simulink model "auto_pilot_udp"  (R2022b)
settings: Solver=FixedStepAuto  StartTime=0.0  StopTime=Inf  FixedStep=0.001  RelTol=1e-3  EnableMultiTasking=on
InitFcn:
  | clear mex
model workspace (MAT data in the model file):
  worldsim_instance : object (value not decoded)
values from neighbouring files (symbols this model uses):
  ACC_Adaptive_D = 0    [AutoPilot_parameters.m]    (also in ap_ini_param.mat; ap_initialModel.sldd = 0.0)
  ACC_Adaptive_I = 0    [AutoPilot_parameters.m]    (also in ap_ini_param.mat; ap_initialModel.sldd = 0.0)
  ACC_Adaptive_P = [5 7.5]    [AutoPilot_parameters.m]    (also in ap_ini_param.mat; ap_initialModel.sldd = 5.0 7.5)
  ACC_Classic_I = 5    [AutoPilot_parameters.m]    (also in ap_ini_param.mat; ap_initialModel.sldd = 5.0)
  ACC_Classic_P = 15    [AutoPilot_parameters.m]    (also in ap_ini_param.mat; ap_initialModel.sldd = 15.0)
  ACC_MaxBrake = 50    [AutoPilot_parameters.m]    (also in ap_ini_param.mat; ap_initialModel.sldd = 50.0)
  ACC_MaxThrottle = 130    [AutoPilot_parameters.m]    (also in ap_ini_param.mat = 80; ap_initialModel.sldd = 130.0)
  ACC_Module_Activity_Flag = 1    [AutoPilot_parameters.m]    (also in ap_ini_param.mat; ap_initialModel.sldd = 1.0)
  ACC_Ready_Speed = 30    [AutoPilot_parameters.m]    (also in ap_ini_param.mat; ap_initialModel.sldd = 30.0)
  ACC_SensorMaxDistance = 250    [AutoPilot_parameters.m]    (also in ap_ini_param.mat = 120; ap_initialModel.sldd = 250.0)
  ACC_Speed_Distance_control = 3    [AutoPilot_parameters.m]    (also in ap_ini_param.mat; ap_initialModel.sldd = 3.0)
  ACC_Speed_Distance_Gain = [0.1 0.15 0.2 0.25]    [AutoPilot_parameters.m]    (also in ap_ini_param.mat; ap_initialModel.sldd = 0.1 0.15 0.2 0.25)
  ADAS_Control_Mode = 1    [AutoPilot_parameters.m]    (also in ap_ini_param.mat; ap_initialModel.sldd = 1.0)
  AEB_Alarm_Freq = 5    [AutoPilot_parameters.m]    (also in ap_ini_param.mat; ap_initialModel.sldd = 5.0)
  AEB_Distance_To_Collision_Brake = 5    [AutoPilot_parameters.m]    (also in ap_ini_param.mat; ap_initialModel.sldd = 5.0)
  AEB_Freq_Hz = Sensor_Freq_worldsim/2    (= 25)    [AutoPilot_parameters.m]    (also in ap_ini_param.mat; ap_initialModel.sldd = 25.0)
  AEB_Gain = [1 1]    [AutoPilot_parameters.m]    (also in ap_ini_param.mat; ap_initialModel.sldd = 1.0 1.0)
  AEB_Gain_set = 60    [AutoPilot_parameters.m]    (also in ap_ini_param.mat; ap_initialModel.sldd = 60.0)
  AEB_Gain_set_mult = 0.03    [AutoPilot_parameters.m]    (also in ap_ini_param.mat; ap_initialModel.sldd)
  AEB_Max_Decel = [8 15]    [AutoPilot_parameters.m]    (also in ap_ini_param.mat; ap_initialModel.sldd = 8.0 15.0)
  AEB_Max_Speed = 150    [AutoPilot_parameters.m]    (also in ap_ini_param.mat = 100; ap_initialModel.sldd = 150.0)
  AEB_Min_Distance_at_Stop = 1    [AutoPilot_parameters.m]    (also in ap_ini_param.mat; ap_initialModel.sldd = 1.0)
  AEB_Module_Activity_Flag = 1    [AutoPilot_parameters.m]    (also in ap_ini_param.mat; ap_initialModel.sldd = 1.0)
  AEB_Pedestrian_type = 68    [AutoPilot_parameters.m]    (also in ap_ini_param.mat; ap_initialModel.sldd = 68.0)
  AEB_Steer_Max = 180    [AutoPilot_parameters.m]    (also in ap_ini_param.mat; ap_initialModel.sldd = 180.0)
  AP_Activity_Flag = 1    [AutoPilot_parameters.m]    (also in ap_ini_param.mat; ap_initialModel.sldd = 1.0)
  AP_D = [0.3 0.3]    [AutoPilot_parameters.m]    (also in ap_ini_param.mat; ap_initialModel.sldd = 0.3 0.3)
  AP_Dyn_Rate_Limiter_Gain = 0.1    [AutoPilot_parameters.m]    (also in ap_ini_param.mat; ap_initialModel.sldd)
  AP_Dyn_Rate_Limiter_Power = 10    [AutoPilot_parameters.m]    (also in ap_ini_param.mat; ap_initialModel.sldd = 10.0)
  AP_Error_Max = 3    [AutoPilot_parameters.m]    (also in ap_ini_param.mat; ap_initialModel.sldd = 3.0)
  AP_Freq_Hz = Sensor_Freq_worldsim    (= 50)    [AutoPilot_parameters.m]    (also in ap_ini_param.mat; ap_initialModel.sldd = 50.0)
  AP_I = [0.05 0.05]    [AutoPilot_parameters.m]    (also in ap_ini_param.mat; ap_initialModel.sldd = 0.05 0.05)
  AP_Max_Error_dydt_Disable = 0.5    [AutoPilot_parameters.m]    (also in ap_ini_param.mat; ap_initialModel.sldd)
  AP_On_Request_Time = 0.01    [AutoPilot_parameters.m]    (also in ap_ini_param.mat; ap_initialModel.sldd)
  AP_P = [0.2 0.2]    [AutoPilot_parameters.m]    (also in ap_ini_param.mat; ap_initialModel.sldd = 0.2 0.2)
  AP_Steer_Error_Max = 0.7    [AutoPilot_parameters.m]    (also in ap_ini_param.mat; ap_initialModel.sldd)
  AP_Steer_Rate_Max_radps = 1    [AutoPilot_parameters.m]    (also in ap_ini_param.mat; ap_initialModel.sldd = 1.0)
  AP_Transition_Rate = 0.5    [AutoPilot_parameters.m]    (also in ap_ini_param.mat; ap_initialModel.sldd)
  butter_a = [1 -1.9911142922 0.991153595869]    [ap_ini_param.mat]    (also in ap_initialModel.sldd = 1.0 -1.9911142922016536 0.99115359586893548)
  butter_a_lka_out = 1.0 -1.5610180758007179 0.641351538057563    [ap_initialModel.sldd]
  butter_b = [9.82591682048e-06 1.9651833641e-05 9.82591682048e-06]    [ap_ini_param.mat]    (also in ap_initialModel.sldd = 9.825916820482009E-6 1.9651833640964018E-5 9.825916820482009)
  butter_b_lka_out = 0.020083365564211246 0.040166731128422492 0.020083365564211246    [ap_initialModel.sldd]
  Lane_Width = 3.7    [AutoPilot_parameters.m]    (also in ap_ini_param.mat; ap_initialModel.sldd)
  LDW_Activity_Flag = 1    [ap_ini_param.mat]    (also in ap_initialModel.sldd = 1.0)
  LDW_Freq_Hz = 50    [ap_ini_param.mat]    (also in ap_initialModel.sldd = 50.0)
  LDW_LaneGap_dydt_Warning = 50    [ap_ini_param.mat]    (also in ap_initialModel.sldd = 50.0)
  LDW_LaneGap_Warning = [0.5 0.25]    [ap_ini_param.mat]    (also in ap_initialModel.sldd = 0.5 0.25)
  LDW_Min_Speed = 60    [ap_ini_param.mat]    (also in ap_initialModel.sldd = 60.0)
  LDW_Steer_Vibration_Amplitude = 5    [ap_ini_param.mat]    (also in ap_initialModel.sldd = 5.0)
  LDW_Steer_Vibration_Freq = 25    [ap_ini_param.mat]    (also in ap_initialModel.sldd = 25.0)
  LKA_Activity_Flag = 1    [ap_ini_param.mat]    (also in ap_initialModel.sldd = 1.0)
  LKA_D = [0.2 0.3]    [ap_ini_param.mat]    (also in ap_initialModel.sldd = 0.2 0.3)
  LKA_Dyn_Rate_Limiter_Gain = 0.1    [ap_ini_param.mat]    (also in ap_initialModel.sldd)
  LKA_Dyn_Rate_Limiter_Power = 10    [ap_ini_param.mat]    (also in ap_initialModel.sldd = 10.0)
  LKA_Error_dydt_Off = 1    [ap_ini_param.mat]    (also in ap_initialModel.sldd = 1.0)
  LKA_Error_Max = 3    [ap_ini_param.mat]    (also in ap_initialModel.sldd = 3.0)
  LKA_Error_Off = 0.5    [ap_ini_param.mat]    (also in ap_initialModel.sldd)
  LKA_Freq_Hz = 50    [ap_ini_param.mat]    (also in ap_initialModel.sldd = 50.0)
  LKA_I = [0.025 0.05]    [ap_ini_param.mat]    (also in ap_initialModel.sldd = 0.025 0.05)
  LKA_Lane_Gap_Activate = [0.25 0.125]    [ap_ini_param.mat]    (also in ap_initialModel.sldd = 0.25 0.125)
  LKA_Lane_Gap_dydt_Activate = 50    [ap_ini_param.mat]    (also in ap_initialModel.sldd = 50.0)
  LKA_Min_Speed = 60    [ap_ini_param.mat]    (also in ap_initialModel.sldd = 60.0)
  LKA_On_Display_Freq = 5    [ap_ini_param.mat]    (also in ap_initialModel.sldd = 5.0)
  LKA_P = [0.1 0.2]    [ap_ini_param.mat]    (also in ap_initialModel.sldd = 0.1 0.2)
  LKA_Steer_Rate_Max_radps = 1    [ap_ini_param.mat]    (also in ap_initialModel.sldd = 1.0)
  No_Target_Display_Value = 0    [AutoPilot_parameters.m]    (also in ap_ini_param.mat; ap_initialModel.sldd = 0.0)
  radar_source = 2    [AutoPilot_parameters.m]    (also in ap_ini_param.mat; ap_initialModel.sldd = 2.0)
  Sensor_Freq_worldsim = 50    [AutoPilot_parameters.m]    (also in ap_ini_param.mat; ap_initialModel.sldd = 50.0; launcher.m)
  stop_number_collisions = 10.0    [ap_initialModel.sldd]    (also in launcher.m = 10)
  stop_speed = 0.001    [ap_initialModel.sldd]    (also in launcher.m)
  stop_time = 12.0    [ap_initialModel.sldd]    (also in launcher.m = 12)
  vehicle_width = 2.2    [AutoPilot_parameters.m]    (also in ap_ini_param.mat = 1.86; ap_initialModel.sldd)
undefined symbols (not defined in the file or in its folder): blockPlatform, HOST, light_brake_center, light_brake_left, light_brake_right
libraries: simulink x103, simwbSfunlib x35, slpidlib x5, viworldsim_lib x5
(part 5 of 5)

== matlab function auto_pilot_udp/OUTPUT/WorldSim_Sensor_Outputs/manipulation_of_objects ==
  data: complete_obstacles_matrix input; filtered_matrix output; detected_objects input
function filtered_matrix = fcn(complete_obstacles_matrix, detected_objects)

% computations

filtered_matrix = complete_obstacles_matrix;

filtered_matrix(:,((detected_objects+1):size(filtered_matrix,2))) = 0;

== matlab function auto_pilot_udp/ACC/ACC_Logic/ACC_Target_Acquisition/SensorTargets_300000_LateralDistance_mux/Target_Lateral_Position ==
  data: Target_distance input; Target_Lateral_Position output; Target_azimuth input
function Target_Lateral_Position = Target_Lateral_Position(Target_distance,Target_azimuth)
%#codegen

Target_Lateral_Position = Target_distance .* sin(Target_azimuth) ;

== matlab function auto_pilot_udp/ACC/ACC_Logic/ACC_Target_Acquisition/SensorTargets_300000_LongitudinalDistance_mux/Target_Longitudinal_Position ==
  data: Target_distance input; Target_Longitudinal_Position output; Target_azimuth input
function Target_Longitudinal_Position = Target_Longitudinal_Position(Target_distance,Target_azimuth)
%#codegen

Target_Longitudinal_Position = Target_distance .* cos(Target_azimuth) ;

== matlab function auto_pilot_udp/AEB/AEB_Logic/MATLAB Function ==
  data: distances_to_collision input; min_distance output
function min_distance = fcn(distances_to_collision)

temp = nonzeros(distances_to_collision);
if isempty(temp)
    min_distance = 121;
else
    min_distance = min(temp);
end

== matlab function auto_pilot_udp/LKA/MATLAB Function ==
  data: u input; y output
function y = fcn(u)

if u == 0
    y=1e-6;
else
    y=u;
end

end

== matlab function auto_pilot_udp/AEB/AEB_Logic/Target_XY_Distance ==
  data: Target_distance_mux input; Target_Y_Distance_mux output; Target_azimuth_mux input; Target_X_Distance_mux output
function [Target_Y_Distance_mux,Target_X_Distance_mux] = Target_XY_Distance(Target_distance_mux,Target_azimuth_mux)
%#codegen

Target_Y_Distance_mux = Target_distance_mux .* sin(Target_azimuth_mux) ;
Target_X_Distance_mux = Target_distance_mux .* cos(Target_azimuth_mux) ;
